simulink model "ModeAdjust"  (R2018b)
settings: Solver=FixedStepDiscrete  StartTime=0.0  StopTime=inf  FixedStep=0.01  RelTol=1e-3
undefined symbols (not defined in the file or in its folder): IfKeSMSbSeatMovBkRclnEnable_Val, IfKeSMSbSeatMovFrwdBkwdEnable_Val, IfKeSMSbSeatMovFtrstEnable_Val, IfKeSMSbSeatMovHdrstFrwdBkwdEnable_Val, IfKeSMSbSeatMovHdUpwdDnwdEnable_Val, IfKeSMSbSeatMovLgrstEnable_Val, IfKeSMSbSeatMovLtwdRtwdEnable_Val, IfVeSMSeStNumConfig, KeSMSbArmscreenMovEnable_Val, KeSMSbSeatMovLgrstExpdEnable_Val, KeSMSuFirstRwStBackPosDelta_Val, KeSMSuFirstRwStBackPosTolr_Val, KeSMSuFirstRwStCushFrntPosDelta_Val, KeSMSuFirstRwStCushFrntPosTolr_Val, KeSMSuFirstRwStCushRePosDelta_Val, KeSMSuFirstRwStCushRePosTolr_Val, KeSMSuFirstRwStFootrestPosDelta_Val, KeSMSuFirstRwStFootrestPosTolr_Val, KeSMSuFirstRwStFwdBkwdPosDelta_Val, KeSMSuFirstRwStFwdBkwdPosTolr_Val, KeSMSuMdMotFinshdTm_Val, KeSMSuMdRetryTm1_Val, KeSMSuModeReqDurgTm_Val, KeSMSuSecRwStArmTochPosDelta_Val, KeSMSuSecRwStArmTochPosTolr_Val, KeSMSuSecRwStBackPosDelta_Val, KeSMSuSecRwStBackPosTolr_Val, KeSMSuSecRwStFtrstUpwdDnwdPosDelta_Val, KeSMSuSecRwStFtrstUpwdDnwdPosTolr_Val, KeSMSuSecRwStFwdBkwdPosDelta_Val, KeSMSuSecRwStFwdBkwdPosTolr_Val, KeSMSuSecRwStHeadrestFwdBkwdPosDelta_Val, KeSMSuSecRwStHeadrestFwdBkwdPosTolr_Val, KeSMSuSecRwStHeadrestUpwdDwnwdPosDelta_Val, KeSMSuSecRwStHeadrestUpwdDwnwdPosTolr_Val, KeSMSuSecRwStLegrestInOutPosDelta_Val, KeSMSuSecRwStLegrestInOutPosTolr_Val, KeSMSuSecRwStLegrestUpwdDwnwdPosDelta_Val, KeSMSuSecRwStLegrestUpwdDwnwdPosTolr_Val, KeSMSuSecRwStLwdRwdPosDelta_Val, KeSMSuSecRwStLwdRwdPosTolr_Val, KeSMSuSecRwStVIPFtrstRefAngle_Val, KeSMSuThirdRwStFwdBkwdPosDelta_Val, KeSMSuThirdRwStFwdBkwdPosTolr_Val, KeSMSuThrdRwCushFoldPosDelta_Val, KeSMSuThrdRwCushFoldPosTolr_Val, KeSMSuThrdRwStBackPosDelta_Val, KeSMSuThrdRwStBackPosTolr_Val, KeSMSw4SLegrstCloseMdSecRwLtStFtrstUpwdDnwdPos_Val, KeSMSw4SLegrstCloseMdSecRwLtStFtrstUpwdDnwdPosMax_Val, KeSMSw4SLegrstCloseMdSecRwLtStFtrstUpwdDnwdPosMin_Val, KeSMSw4SLegrstCloseMdSecRwLtStLgrstOtwdInwdPos_Val, KeSMSw4SLegrstCloseMdSecRwLtStLgrstOtwdInwdPosMax_Val, KeSMSw4SLegrstCloseMdSecRwLtStLgrstOtwdInwdPosMin_Val, KeSMSw4SLegrstCloseMdSecRwLtStLgrstUpwdDnwdPos_Val, KeSMSw4SLegrstCloseMdSecRwLtStLgrstUpwdDnwdPosMax_Val, KeSMSw4SLegrstCloseMdSecRwLtStLgrstUpwdDnwdPosMin_Val, KeSMSw4SLegrstCloseMdSecRwRtStFtrstUpwdDnwdPos_Val, KeSMSw4SLegrstCloseMdSecRwRtStFtrstUpwdDnwdPosMax_Val, KeSMSw4SLegrstCloseMdSecRwRtStFtrstUpwdDnwdPosMin_Val ... (+1138)
libraries: Lib x401
(part 14 of 35)

== system ModeAdjust/ModeAdjustRunnable_sys/ModeAdjust/ArrivedAtTargetPosChk/INTMR ==
  SecRwLtStsPoss : Inport
  SecRwRtStPoss : Inport  Port=2
  ModeStCalib : Inport  Port=3
  StConfig : Inport  Port=4
  SecRwLtStsPossV : Inport  Port=5
  SecRwRtStPossV : Inport  Port=6
  PosDeltaCalib : Inport  Port=7
  Bus Selector : BusSelector  OutputSignals=Calib_Drv,Calib_Pass,Calib_2L,Calib_2R,Calib_3L,Calib_3R
  Bus Selector1 : BusSelector  OutputSignals=DrvStConfig,PassStConfig,SecRwLtStConfig,SecRwRtStConfig,ThdRwLtStConfig,ThdRwRtStConfig
  Logical Operator : Logic  AllPortsSameDT=off  OutDataTypeStr=boolean
  R2Lt : Subsystem
  R2Rt : Subsystem
  isINTMArrivedAtTargetPos : Outport
  wires:
  SecRwRtStPossV/1 -> R2Rt/4(SecRwRtStPossV)
  SecRwLtStsPossV/1 -> R2Lt/4(SecRwLtStPossV)
  [R2RtST_ArrivedTarPos] -> Logical Operator/2
  [R2LtST_ArrivedTarPos] -> Logical Operator/1
  Logical Operator/1 -> isINTMArrivedAtTargetPos/1
  R2Lt/1(R2Lt_ArrivedTarPos) -> [R2LtST_ArrivedTarPos]
  R2Rt/1(R2Rt_ArrivedTarPos) -> [R2RtST_ArrivedTarPos]
  SecRwLtStsPoss/1 -> R2Rt/5(SecRwLtStsPoss), R2Lt/1(SecRwLtStsPoss)
  SecRwRtStPoss/1 -> R2Rt/1(SecRwRtStPoss)
  Bus Selector/6 -> [ModeStCalib_3R]  "<Calib_3R>"
  Bus Selector/4 -> [ModeStCalib_2R]  "<Calib_2R>"
  Bus Selector/1 -> [ModeStCalib_Drv]  "<Calib_Drv>"
  Bus Selector/3 -> [ModeStCalib_2L]  "<Calib_2L>"
  Bus Selector/5 -> [ModeStCalib_3L]  "<Calib_3L>"
  Bus Selector/2 -> [ModeStCalib_Pass]  "<Calib_Pass>"
  ModeStCalib/1 -> Bus Selector/1
  [ModeStCalib_2R] -> R2Rt/2(ModeStCalib_2R)
  [ModeStCalib_2L] -> R2Lt/2(ModeStCalib_2L)
  Bus Selector1/6 -> [ThdRwRtStConfig]  "<ThdRwRtStConfig>"
  Bus Selector1/1 -> [DrvStConfig]  "<DrvStConfig>"
  Bus Selector1/3 -> [SecRwLtStConfig]  "<SecRwLtStConfig>"
  Bus Selector1/4 -> [SecRwRtStConfig]  "<SecRwRtStConfig>"
  StConfig/1 -> Bus Selector1/1
  Bus Selector1/2 -> [PassStConfig]  "<PassStConfig>"
  Bus Selector1/5 -> [ThdRwLtStConfig]  "<ThdRwLtStConfig>"
  [SecRwLtStConfig] -> R2Lt/3(StConfig)
  [SecRwRtStConfig] -> R2Rt/3(StConfig)
  PosDeltaCalib/1 -> [PosDeltaCalib]
  [PosDeltaCalib] -> R2Lt/5(PosDeltaCalib)
  [PosDeltaCalib] -> R2Rt/6(PosDeltaCalib)

== system ModeAdjust/ModeAdjustRunnable_sys/ModeAdjust/ArrivedAtTargetPosChk/LgrstClose ==
  SecRwLtStsPoss : Inport
  SecRwRtStPoss : Inport  Port=2
  ModeStCalib : Inport  Port=3
  StConfig : Inport  Port=4
  SecRwLtStsPoss4s : Inport  Port=5
  SecRwRtStsPoss4s : Inport  Port=6
  StConfig4s : Inport  Port=7
  SecRwLtStsPossV : Inport  Port=8
  SecRwRtStPossV : Inport  Port=9
  SecRwLtStsPoss4sV : Inport  Port=10
  SecRwRtStsPoss4sV : Inport  Port=11
  PosDeltaCalib : Inport  Port=12
  Bus Selector : BusSelector  OutputSignals=Calib_Drv,Calib_Pass,Calib_2L,Calib_2R,Calib_3L,Calib_3R,Calib_2L4s,Calib_2R4s
  Bus Selector1 : BusSelector  OutputSignals=DrvStConfig,PassStConfig,SecRwLtStConfig,SecRwRtStConfig,ThdRwLtStConfig,ThdRwRtStConfig
  Bus Selector5 : BusSelector  OutputSignals=SecRwLtStConfig,SecRwRtStConfig
  R2Lt : Subsystem
  R2Rt : Subsystem
  isLfRecoveryArrivedAtTargetPos : Outport
  isRtRecoveryArrivedAtTargetPos : Outport  Port=2
  wires:
  SecRwLtStsPoss4sV/1 -> R2Lt/7(SecRwLtStPossV4s)
  SecRwRtStsPoss4sV/1 -> R2Rt/7(PosV4s)
  SecRwRtStPossV/1 -> R2Rt/6(SecRwRtStPossV)
  SecRwLtStsPossV/1 -> R2Lt/6(SecRwLtStPossV)
  [R2LtST_ArrivedTarPos] -> isLfRecoveryArrivedAtTargetPos/1
  R2Lt/1(R2Lt_ArrivedTarPos) -> [R2LtST_ArrivedTarPos]
  R2Rt/1(R2Lt_ArrivedTarPos) -> [R2RtST_ArrivedTarPos]
  SecRwLtStsPoss/1 -> R2Lt/1(SecRwLtStsPoss)
  SecRwRtStPoss/1 -> R2Rt/1(SecRwLtStsPoss)
  [R2RtST_ArrivedTarPos] -> isRtRecoveryArrivedAtTargetPos/1
  Bus Selector/6 -> [ModeStCalib_3R]  "<Calib_3R>"
  Bus Selector/4 -> [ModeStCalib_2R]  "<Calib_2R>"
  Bus Selector/1 -> [ModeStCalib_Drv]  "<Calib_Drv>"
  Bus Selector/3 -> [ModeStCalib_2L]  "<Calib_2L>"
  Bus Selector/5 -> [ModeStCalib_3L]  "<Calib_3L>"
  Bus Selector/2 -> [ModeStCalib_Pass]  "<Calib_Pass>"
  ModeStCalib/1 -> Bus Selector/1
  [Calib_2R4s] -> R2Rt/2(ModeStCalib_2L)
  [Calib_2L4s] -> R2Lt/2(ModeStCalib_2L)
  Bus Selector1/6 -> [ThdRwRtStConfig]  "<ThdRwRtStConfig>"
  Bus Selector1/1 -> [DrvStConfig]  "<DrvStConfig>"
  Bus Selector1/3 -> [SecRwLtStConfig]  "<SecRwLtStConfig>"
  Bus Selector1/4 -> [SecRwRtStConfig]  "<SecRwRtStConfig>"
  StConfig/1 -> Bus Selector1/1
  Bus Selector1/2 -> [PassStConfig]  "<PassStConfig>"
  Bus Selector1/5 -> [ThdRwLtStConfig]  "<ThdRwLtStConfig>"
  [SecRwLtStConfig] -> R2Lt/3(StConfig)
  [SecRwRtStConfig] -> R2Rt/3(StConfig)
  Bus Selector/8 -> [Calib_2R4s]  "<Calib_2R4s>"
  Bus Selector/7 -> [Calib_2L4s]  "<Calib_2L4s>"
  SecRwLtStsPoss4s/1 -> R2Lt/4(SecRwLtStsPoss4s)
  SecRwRtStsPoss4s/1 -> R2Rt/4(SecRwLtStsPoss4s)
  StConfig4s/1 -> Bus Selector5/1
  Bus Selector5/1 -> [SecRwLtStConfig4s]  "<SecRwLtStConfig>"
  Bus Selector5/2 -> [SecRwRtStConfig4s]  "<SecRwRtStConfig>"
  [SecRwLtStConfig4s] -> R2Lt/5(StConfig4s)
  [SecRwRtStConfig4s] -> R2Rt/5(StConfig4s)
  PosDeltaCalib/1 -> [PosDeltaCalib]
  [PosDeltaCalib] -> R2Lt/8(PosDeltaCalib)
  [PosDeltaCalib] -> R2Rt/8(PosDeltaCalib)

== system ModeAdjust/ModeAdjustRunnable_sys/ModeAdjust/ArrivedAtTargetPosChk/LgrstOpen ==
  SecRwLtStsPoss : Inport
  SecRwRtStPoss : Inport  Port=2
  ModeStCalib : Inport  Port=3
  StConfig : Inport  Port=4
  SecRwLtStsPoss4s : Inport  Port=5
  SecRwRtStsPoss4s : Inport  Port=6
  StConfig4s : Inport  Port=7
  SecRwLtStsPossV : Inport  Port=8
  SecRwRtStPossV : Inport  Port=9
  SecRwLtStsPoss4sV : Inport  Port=10
  SecRwRtStsPoss4sV : Inport  Port=11
  PosDeltaCalib : Inport  Port=12
  Bus Selector : BusSelector  OutputSignals=Calib_Drv,Calib_Pass,Calib_2L,Calib_2R,Calib_3L,Calib_3R,Calib_2L4s,Calib_2R4s
  Bus Selector1 : BusSelector  OutputSignals=DrvStConfig,PassStConfig,SecRwLtStConfig,SecRwRtStConfig,ThdRwLtStConfig,ThdRwRtStConfig
  Bus Selector5 : BusSelector  OutputSignals=SecRwLtStConfig,SecRwRtStConfig
  R2Lt : Subsystem
  R2Rt : Subsystem
  isLfRecoveryArrivedAtTargetPos : Outport
  isRtRecoveryArrivedAtTargetPos : Outport  Port=2
  wires:
  [SecRwRtStConfig4s] -> R2Rt/5(StConfig4s)
  [SecRwLtStConfig4s] -> R2Lt/5(StConfig4s)
  Bus Selector5/2 -> [SecRwRtStConfig4s]  "<SecRwRtStConfig>"
  Bus Selector5/1 -> [SecRwLtStConfig4s]  "<SecRwLtStConfig>"
  StConfig4s/1 -> Bus Selector5/1
  SecRwRtStsPoss4s/1 -> R2Rt/4(SecRwLtStsPoss4s)
  SecRwLtStsPoss4s/1 -> R2Lt/4(SecRwLtStsPoss4s)
  Bus Selector/7 -> [Calib_2L4s]  "<Calib_2L4s>"
  Bus Selector/8 -> [Calib_2R4s]  "<Calib_2R4s>"
  [SecRwRtStConfig] -> R2Rt/3(StConfig)
  [SecRwLtStConfig] -> R2Lt/3(StConfig)
  Bus Selector1/5 -> [ThdRwLtStConfig]  "<ThdRwLtStConfig>"
  Bus Selector1/2 -> [PassStConfig]  "<PassStConfig>"
  StConfig/1 -> Bus Selector1/1
  Bus Selector1/4 -> [SecRwRtStConfig]  "<SecRwRtStConfig>"
  Bus Selector1/3 -> [SecRwLtStConfig]  "<SecRwLtStConfig>"
  Bus Selector1/1 -> [DrvStConfig]  "<DrvStConfig>"
  Bus Selector1/6 -> [ThdRwRtStConfig]  "<ThdRwRtStConfig>"
  [Calib_2L4s] -> R2Lt/2(ModeStCalib_2L)
  [Calib_2R4s] -> R2Rt/2(ModeStCalib_2L)
  ModeStCalib/1 -> Bus Selector/1
  Bus Selector/2 -> [ModeStCalib_Pass]  "<Calib_Pass>"
  Bus Selector/5 -> [ModeStCalib_3L]  "<Calib_3L>"
  Bus Selector/3 -> [ModeStCalib_2L]  "<Calib_2L>"
  Bus Selector/1 -> [ModeStCalib_Drv]  "<Calib_Drv>"
  Bus Selector/4 -> [ModeStCalib_2R]  "<Calib_2R>"
  Bus Selector/6 -> [ModeStCalib_3R]  "<Calib_3R>"
  [R2RtST_ArrivedTarPos] -> isRtRecoveryArrivedAtTargetPos/1
  SecRwRtStPoss/1 -> R2Rt/1(SecRwLtStsPoss)
  SecRwLtStsPoss/1 -> R2Lt/1(SecRwLtStsPoss)
  R2Rt/1(R2Lt_ArrivedTarPos) -> [R2RtST_ArrivedTarPos]
  R2Lt/1(R2Lt_ArrivedTarPos) -> [R2LtST_ArrivedTarPos]
  [R2LtST_ArrivedTarPos] -> isLfRecoveryArrivedAtTargetPos/1
  SecRwLtStsPossV/1 -> R2Lt/6(SecRwLtStPossV)
  SecRwLtStsPoss4sV/1 -> R2Lt/7(SecRwLtStPossV4s)
  SecRwRtStPossV/1 -> R2Rt/6(SecRwRtStPossV)
  SecRwRtStsPoss4sV/1 -> R2Rt/7(PosV4s)
  PosDeltaCalib/1 -> [PosDeltaCalib]
  [PosDeltaCalib] -> R2Lt/8(PosDeltaCalib)
  [PosDeltaCalib] -> R2Rt/8(PosDeltaCalib)

== system ModeAdjust/ModeAdjustRunnable_sys/ModeAdjust/ArrivedAtTargetPosChk/Lug ==
  ThdRwLtStPoss : Inport
  ThdRwRtStPoss : Inport  Port=2
  ModeStCalib : Inport  Port=3
  is6s : Inport  Port=4
  StConfig : Inport  Port=5
  IfVeSMSbThdRwLtStFrwdCmdSrv_Val_read : Inport  Port=6
  IfVeSMSbThdRwRtStFrwdCmdSrv_Val_read : Inport  Port=7
  ThdRwLtStPossV : Inport  Port=8
  ThdRwRtStPossV : Inport  Port=9
  PosDeltaCalib : Inport  Port=10
  Bus Selector : BusSelector  OutputSignals=Calib_Drv,Calib_Pass,Calib_2L,Calib_2R,Calib_3L,Calib_3R
  Bus Selector1 : BusSelector  OutputSignals=DrvStConfig,PassStConfig,SecRwLtStConfig,SecRwRtStConfig,ThdRwLtStConfig,ThdRwRtStConfig
  R3Lt : Subsystem
  R3Rt : Subsystem
  Subsystem1 : Subsystem
  isLfLugArrivedAtTargetPos : Outport
  isRtLugArrivedAtTargetPos : Outport  Port=2
  wires:
  ThdRwRtStPoss/1 -> R3Rt/1(ThdRwRtStPoss)
  ThdRwLtStPoss/1 -> R3Lt/1(ThdRwLtStPoss)
  R3Rt/1(R3Rt_ArrivedTarPos) -> [R3RtST_ArrivedTarPos]
  R3Lt/1(R3Lt_ArrivedTarPos) -> [R3LtST_ArrivedTarPos]
  Subsystem1/1(Md_L_MvDoneOK) -> isLfLugArrivedAtTargetPos/1
  [R3LtST_ArrivedTarPos] -> Subsystem1/1(Left_inport)
  [R3RtST_ArrivedTarPos] -> Subsystem1/2(Right_inport)
  Subsystem1/2(Md_R_MvDoneOK) -> isRtLugArrivedAtTargetPos/1
  Bus Selector/6 -> [ModeStCalib_3R]  "<Calib_3R>"
  Bus Selector/4 -> [ModeStCalib_2R]  "<Calib_2R>"
  Bus Selector/1 -> [ModeStCalib_Drv]  "<Calib_Drv>"
  Bus Selector/3 -> [ModeStCalib_2L]  "<Calib_2L>"
  Bus Selector/5 -> [ModeStCalib_3L]  "<Calib_3L>"
  Bus Selector/2 -> [ModeStCalib_Pass]  "<Calib_Pass>"
  ModeStCalib/1 -> Bus Selector/1
  [ModeStCalib_3L] -> R3Lt/2(ModeStCalib_3L)
  [ModeStCalib_3R] -> R3Rt/2(ModeStCalib_3R)
  is6s/1 -> [is6s]
  [is6s] -> R3Lt/3(is6s)
  [is6s] -> R3Rt/3(is6s)
  Bus Selector1/6 -> [ThdRwRtStConfig]  "<ThdRwRtStConfig>"
  Bus Selector1/1 -> [DrvStConfig]  "<DrvStConfig>"
  Bus Selector1/3 -> [SecRwLtStConfig]  "<SecRwLtStConfig>"
  Bus Selector1/4 -> [SecRwRtStConfig]  "<SecRwRtStConfig>"
  StConfig/1 -> Bus Selector1/1
  Bus Selector1/2 -> [PassStConfig]  "<PassStConfig>"
  Bus Selector1/5 -> [ThdRwLtStConfig]  "<ThdRwLtStConfig>"
  [ThdRwLtStConfig] -> R3Lt/4(StConfig)
  [ThdRwRtStConfig] -> R3Rt/4(StConfig)
  IfVeSMSbThdRwLtStFrwdCmdSrv_Val_read/1 -> R3Lt/5(IfVeSMSbThdRwLtStFrwdCmdSrv_Val_read)
  IfVeSMSbThdRwRtStFrwdCmdSrv_Val_read/1 -> R3Rt/5(IfVeSMSbThdRwRtStFrwdCmdSrv_Val_read)
  ThdRwLtStPossV/1 -> R3Lt/6(ThdRwLtStPossV)
  ThdRwRtStPossV/1 -> R3Rt/6(ThdRwRtStPossV)
  PosDeltaCalib/1 -> [PosDeltaCalib]
  [PosDeltaCalib] -> R3Lt/7(PosDeltaCalib)
  [PosDeltaCalib] -> R3Rt/7(PosDeltaCalib)

== system ModeAdjust/ModeAdjustRunnable_sys/ModeAdjust/ArrivedAtTargetPosChk/Ly ==
  SecRwLtStsPoss : Inport
  SecRwRtStPoss : Inport  Port=2
  ModeStCalib : Inport  Port=3
  StConfig : Inport  Port=4
  SecRwLtStsPoss4s : Inport  Port=5
  SecRwRtStsPoss4s : Inport  Port=6
  StConfig4s : Inport  Port=7
  SecRwLtStsPossV : Inport  Port=8
  SecRwRtStPossV : Inport  Port=9
  SecRwLtStsPoss4sV : Inport  Port=10
  SecRwRtStsPoss4sV : Inport  Port=11
  Lt4sHightIndex : Inport  Port=12
  Rt4sHightIndex : Inport  Port=13
  PosDeltaCalib : Inport  Port=14
  Bus Selector : BusSelector  OutputSignals=Calib_Drv,Calib_Pass,Calib_2L,Calib_2R,Calib_3L,Calib_3R,Calib_2L4s,Calib_2R4s
  Bus Selector1 : BusSelector  OutputSignals=DrvStConfig,PassStConfig,SecRwLtStConfig,SecRwRtStConfig,ThdRwLtStConfig,ThdRwRtStConfig
  Bus Selector5 : BusSelector  OutputSignals=SecRwLtStConfig,SecRwRtStConfig
  R2Lt : Subsystem
  R2Rt : Subsystem
  isLfRecoveryArrivedAtTargetPos : Outport
  isRtRecoveryArrivedAtTargetPos : Outport  Port=2
  Calib_Ly4sLAdpt : Outport  Port=3
  Calib_Ly4sRAdpt : Outport  Port=4
  wires:
  [R2LtST_ArrivedTarPos] -> isLfRecoveryArrivedAtTargetPos/1
  R2Lt/1(R2Lt_ArrivedTarPos) -> [R2LtST_ArrivedTarPos]
  R2Rt/1(R2Lt_ArrivedTarPos) -> [R2RtST_ArrivedTarPos]
  SecRwLtStsPoss/1 -> R2Lt/1(SecRwLtStsPoss)
  SecRwRtStPoss/1 -> R2Rt/1(SecRwLtStsPoss)
  [R2RtST_ArrivedTarPos] -> isRtRecoveryArrivedAtTargetPos/1
  Bus Selector/6 -> [ModeStCalib_3R]  "<Calib_3R>"
  Bus Selector/4 -> [ModeStCalib_2R]  "<Calib_2R>"
  Bus Selector/1 -> [ModeStCalib_Drv]  "<Calib_Drv>"
  Bus Selector/3 -> [ModeStCalib_2L]  "<Calib_2L>"
  Bus Selector/5 -> [ModeStCalib_3L]  "<Calib_3L>"
  Bus Selector/2 -> [ModeStCalib_Pass]  "<Calib_Pass>"
  ModeStCalib/1 -> Bus Selector/1
  [Calib_2R4s] -> R2Rt/2(ModeStCalib_2L)
  [Calib_2L4s] -> R2Lt/2(ModeStCalib_2L)
  Bus Selector1/6 -> [ThdRwRtStConfig]  "<ThdRwRtStConfig>"
  Bus Selector1/1 -> [DrvStConfig]  "<DrvStConfig>"
  Bus Selector1/3 -> [SecRwLtStConfig]  "<SecRwLtStConfig>"
  Bus Selector1/4 -> [SecRwRtStConfig]  "<SecRwRtStConfig>"
  StConfig/1 -> Bus Selector1/1
  Bus Selector1/2 -> [PassStConfig]  "<PassStConfig>"
  Bus Selector1/5 -> [ThdRwLtStConfig]  "<ThdRwLtStConfig>"
  [SecRwLtStConfig] -> R2Lt/3(StConfig)
  [SecRwRtStConfig] -> R2Rt/3(StConfig)
  Bus Selector/8 -> [Calib_2R4s]  "<Calib_2R4s>"
  Bus Selector/7 -> [Calib_2L4s]  "<Calib_2L4s>"
  SecRwLtStsPoss4s/1 -> R2Lt/4(SecRwLtStsPoss4s)
  SecRwRtStsPoss4s/1 -> R2Rt/4(SecRwLtStsPoss4s)
  StConfig4s/1 -> Bus Selector5/1
  Bus Selector5/1 -> [SecRwLtStConfig4s]  "<SecRwLtStConfig>"
  Bus Selector5/2 -> [SecRwRtStConfig4s]  "<SecRwRtStConfig>"
  [SecRwLtStConfig4s] -> R2Lt/5(StConfig4s)
  [SecRwRtStConfig4s] -> R2Rt/5(StConfig4s)
  SecRwLtStsPoss4sV/1 -> R2Lt/7(SecRwLtStPossV4s)
  SecRwRtStsPoss4sV/1 -> R2Rt/7(PosV4s)
  SecRwLtStsPossV/1 -> R2Lt/6(SecRwLtStPossV)
  SecRwRtStPossV/1 -> R2Rt/6(SecRwRtStPossV)
  Lt4sHightIndex/1 -> R2Lt/8(Lt4sHightIndex)
  Rt4sHightIndex/1 -> R2Rt/8(Rt4sHightIndex)
  R2Lt/2(Calib_Ly4sLAdpt) -> Calib_Ly4sLAdpt/1
  R2Rt/2(Calib_Ly4sRAdpt) -> Calib_Ly4sRAdpt/1
  PosDeltaCalib/1 -> [PosDeltaCalib]
  [PosDeltaCalib] -> R2Lt/9(PosDeltaCalib)
  [PosDeltaCalib] -> R2Rt/9(PosDeltaCalib)

== system ModeAdjust/ModeAdjustRunnable_sys/ModeAdjust/ArrivedAtTargetPosChk/Recovery ==
  SecRwLtStsPoss : Inport
  SecRwRtStPoss : Inport  Port=2
  ModeStCalib : Inport  Port=3
  StConfig : Inport  Port=4
  DrvCurPos : Inport  Port=5
  PassStPoss : Inport  Port=6
  DrvCurPosV : Inport  Port=7
  PassStPossV : Inport  Port=8
  SecRwLtStsPossV : Inport  Port=9
  SecRwRtStPossV : Inport  Port=10
  PosDeltaCalib : Inport  Port=11
  Bus Selector : BusSelector  OutputSignals=Calib_Drv,Calib_Pass,Calib_2L,Calib_2R,Calib_3L,Calib_3R
  Bus Selector1 : BusSelector  OutputSignals=DrvStConfig,PassStConfig,SecRwLtStConfig,SecRwRtStConfig,ThdRwLtStConfig,ThdRwRtStConfig
  Drv : Subsystem
  Logical Operator : Logic  AllPortsSameDT=off  OutDataTypeStr=boolean
  Logical Operator1 : Logic  AllPortsSameDT=off  OutDataTypeStr=boolean
  Pass : Subsystem
  R2Lt : Subsystem
  R2Rt : Subsystem
  isLfRecoveryArrivedAtTargetPos : Outport
  isRtRecoveryArrivedAtTargetPos : Outport  Port=2
  wires:
  Logical Operator/1 -> isLfRecoveryArrivedAtTargetPos/1
  R2Lt/1(R2Lt_ArrivedTarPos) -> [R2LtST_ArrivedTarPos]
  R2Rt/1(R2Rt_ArrivedTarPos) -> [R2RtST_ArrivedTarPos]
  SecRwLtStsPoss/1 -> R2Lt/1(SecRwLtStsPoss)
  SecRwRtStPoss/1 -> R2Rt/1(SecRwRtStPoss)
  Logical Operator1/1 -> isRtRecoveryArrivedAtTargetPos/1
  Bus Selector/6 -> [ModeStCalib_3R]  "<Calib_3R>"
  Bus Selector/4 -> [ModeStCalib_2R]  "<Calib_2R>"
  Bus Selector/1 -> [ModeStCalib_Drv]  "<Calib_Drv>"
  Bus Selector/3 -> [ModeStCalib_2L]  "<Calib_2L>"
  Bus Selector/5 -> [ModeStCalib_3L]  "<Calib_3L>"
  Bus Selector/2 -> [ModeStCalib_Pass]  "<Calib_Pass>"
  ModeStCalib/1 -> Bus Selector/1
  [ModeStCalib_2R] -> R2Rt/2(ModeStCalib_2R)
  [ModeStCalib_2L] -> R2Lt/2(ModeStCalib_2L)
  Bus Selector1/6 -> [ThdRwRtStConfig]  "<ThdRwRtStConfig>"
  Bus Selector1/1 -> [DrvStConfig]  "<DrvStConfig>"
  Bus Selector1/3 -> [SecRwLtStConfig]  "<SecRwLtStConfig>"
  Bus Selector1/4 -> [SecRwRtStConfig]  "<SecRwRtStConfig>"
  StConfig/1 -> Bus Selector1/1
  Bus Selector1/2 -> [PassStConfig]  "<PassStConfig>"
  Bus Selector1/5 -> [ThdRwLtStConfig]  "<ThdRwLtStConfig>"
  [SecRwLtStConfig] -> R2Lt/3(StConfig)
  [SecRwRtStConfig] -> R2Rt/3(StConfig)
  Drv/1(Drv_ArrivedTarPos) -> [DrvST_ArrivedTarPos]
  [DrvStConfig] -> Drv/3(StConfig)
  DrvCurPos/1 -> Drv/1(DrvCurPos)
  [ModeStCalib_Drv] -> Drv/2(ModeStCalib_Drv)
  Pass/1(Pass_ArrivedTarPos) -> [Pass_ArrivedTarPos]
  [ModeStCalib_Pass] -> Pass/2(ModeStCalib_Pass)
  PassStPoss/1 -> Pass/1(PassStPoss)
  [PassStConfig] -> Pass/3(StConfig)
  [R2LtST_ArrivedTarPos] -> Logical Operator/1
  [DrvST_ArrivedTarPos] -> Logical Operator/2
  [R2RtST_ArrivedTarPos] -> Logical Operator1/1
  [Pass_ArrivedTarPos] -> Logical Operator1/2
  DrvCurPosV/1 -> Drv/4(DrvCurPosV)
  PassStPossV/1 -> Pass/4(PassStPossV)
  SecRwLtStsPossV/1 -> R2Lt/4(SecRwLtStPossV)
  SecRwRtStPossV/1 -> R2Rt/4(SecRwRtStPossV)
  PosDeltaCalib/1 -> [PosDeltaCalib]
  [PosDeltaCalib] -> Drv/5(PosDeltaCalib)
  [PosDeltaCalib] -> Pass/5(PosDeltaCalib)
  [PosDeltaCalib] -> R2Lt/5(PosDeltaCalib)
  [PosDeltaCalib] -> R2Rt/5(PosDeltaCalib)

== system ModeAdjust/ModeAdjustRunnable_sys/ModeAdjust/ArrivedAtTargetPosChk/Recovery4s ==
  SecRwLtStsPoss : Inport
  SecRwRtStPoss : Inport  Port=2
  ModeStCalib : Inport  Port=3
  StConfig : Inport  Port=4
  SecRwLtStsPoss4s : Inport  Port=5
  SecRwRtStsPoss4s : Inport  Port=6
  StConfig4s : Inport  Port=7
  SecRwLtStsPossV : Inport  Port=8
  SecRwRtStPossV : Inport  Port=9
  SecRwLtStsPoss4sV : Inport  Port=10
  SecRwRtStsPoss4sV : Inport  Port=11
  Lt4sHightIndex : Inport  Port=12
  Rt4sHightIndex : Inport  Port=13
  PosDeltaCalib : Inport  Port=14
  Bus Selector : BusSelector  OutputSignals=Calib_Drv,Calib_Pass,Calib_2L,Calib_2R,Calib_3L,Calib_3R,Calib_2L4s,Calib_2R4s
  Bus Selector1 : BusSelector  OutputSignals=DrvStConfig,PassStConfig,SecRwLtStConfig,SecRwRtStConfig,ThdRwLtStConfig,ThdRwRtStConfig
  Bus Selector5 : BusSelector  OutputSignals=SecRwLtStConfig,SecRwRtStConfig
  R2Lt : Subsystem
  R2Rt : Subsystem
  isLfRecoveryArrivedAtTargetPos : Outport
  isRtRecoveryArrivedAtTargetPos : Outport  Port=2
  Calib_Recoery4sLAdpt : Outport  Port=3
  Calib_Recoery4sRAdpt : Outport  Port=4
  wires:
  [SecRwRtStConfig4s] -> R2Rt/5(StConfig4s)
  [SecRwLtStConfig4s] -> R2Lt/5(StConfig4s)
  Bus Selector5/2 -> [SecRwRtStConfig4s]  "<SecRwRtStConfig>"
  Bus Selector5/1 -> [SecRwLtStConfig4s]  "<SecRwLtStConfig>"
  StConfig4s/1 -> Bus Selector5/1
  SecRwRtStsPoss4s/1 -> R2Rt/4(SecRwLtStsPoss4s)
  SecRwLtStsPoss4s/1 -> R2Lt/4(SecRwLtStsPoss4s)
  Bus Selector/7 -> [Calib_2L4s]  "<Calib_2L4s>"
  Bus Selector/8 -> [Calib_2R4s]  "<Calib_2R4s>"
  [SecRwRtStConfig] -> R2Rt/3(StConfig)
  [SecRwLtStConfig] -> R2Lt/3(StConfig)
  Bus Selector1/5 -> [ThdRwLtStConfig]  "<ThdRwLtStConfig>"
  Bus Selector1/2 -> [PassStConfig]  "<PassStConfig>"
  StConfig/1 -> Bus Selector1/1
  Bus Selector1/4 -> [SecRwRtStConfig]  "<SecRwRtStConfig>"
  Bus Selector1/3 -> [SecRwLtStConfig]  "<SecRwLtStConfig>"
  Bus Selector1/1 -> [DrvStConfig]  "<DrvStConfig>"
  Bus Selector1/6 -> [ThdRwRtStConfig]  "<ThdRwRtStConfig>"
  [Calib_2L4s] -> R2Lt/2(ModeStCalib_2L)
  [Calib_2R4s] -> R2Rt/2(ModeStCalib_2L)
  ModeStCalib/1 -> Bus Selector/1
  Bus Selector/2 -> [ModeStCalib_Pass]  "<Calib_Pass>"
  Bus Selector/5 -> [ModeStCalib_3L]  "<Calib_3L>"
  Bus Selector/3 -> [ModeStCalib_2L]  "<Calib_2L>"
  Bus Selector/1 -> [ModeStCalib_Drv]  "<Calib_Drv>"
  Bus Selector/4 -> [ModeStCalib_2R]  "<Calib_2R>"
  Bus Selector/6 -> [ModeStCalib_3R]  "<Calib_3R>"
  [R2RtST_ArrivedTarPos] -> isRtRecoveryArrivedAtTargetPos/1
  SecRwRtStPoss/1 -> R2Rt/1(SecRwLtStsPoss)
  SecRwLtStsPoss/1 -> R2Lt/1(SecRwLtStsPoss)
  R2Rt/1(R2Lt_ArrivedTarPos) -> [R2RtST_ArrivedTarPos]
  R2Lt/1(R2Lt_ArrivedTarPos) -> [R2LtST_ArrivedTarPos]
  [R2LtST_ArrivedTarPos] -> isLfRecoveryArrivedAtTargetPos/1
  SecRwLtStsPossV/1 -> R2Lt/6(SecRwLtStPossV)
  SecRwRtStPossV/1 -> R2Rt/6(SecRwRtStPossV)
  SecRwRtStsPoss4sV/1 -> R2Rt/7(PosV4s)
  SecRwLtStsPoss4sV/1 -> R2Lt/7(SecRwLtStPossV4s)
  Lt4sHightIndex/1 -> R2Lt/8(Lt4sHightIndex)
  Rt4sHightIndex/1 -> R2Rt/8(Rt4sHightIndex)
  R2Lt/2(Calib_Recoery4sLAdpt) -> Calib_Recoery4sLAdpt/1
  R2Rt/2(Calib_Recoery4sRAdpt) -> Calib_Recoery4sRAdpt/1
  PosDeltaCalib/1 -> [PosDeltaCalib]
  [PosDeltaCalib] -> R2Lt/9(PosDeltaCalib)
  [PosDeltaCalib] -> R2Rt/9(PosDeltaCalib)

== system ModeAdjust/ModeAdjustRunnable_sys/ModeAdjust/ArrivedAtTargetPosChk/VIP ==
  SecRwLtStsPoss : Inport
  SecRwRtStPoss : Inport  Port=2
  ThdRwLtStPoss : Inport  Port=3
  ThdRwRtStPoss : Inport  Port=4
  ModeStCalib : Inport  Port=5
  is6s : Inport  Port=6
  StConfig : Inport  Port=7
  DrvCurPos : Inport  Port=8
  PassStPoss : Inport  Port=9
  DrvCurPosV : Inport  Port=10
  PassStPossV : Inport  Port=11
  SecRwLtStsPossV : Inport  Port=12
  SecRwRtStPossV : Inport  Port=13
  ThdRwLtStPossV : Inport  Port=14
  ThdRwRtStPossV : Inport  Port=15
  PosDeltaCalib : Inport  Port=16
  Bus Selector : BusSelector  OutputSignals=Calib_Drv,Calib_Pass,Calib_2L,Calib_2R,Calib_3L,Calib_3R
  Bus Selector1 : BusSelector  OutputSignals=DrvStConfig,PassStConfig,SecRwLtStConfig,SecRwRtStConfig,ThdRwLtStConfig,ThdRwRtStConfig
  Drv : Subsystem
  Logical Operator1 : Logic  Inputs=3  AllPortsSameDT=off  OutDataTypeStr=boolean
  Logical Operator3 : Logic  Operator=OR  AllPortsSameDT=off  OutDataTypeStr=boolean
  Logical Operator7 : Logic  Inputs=4  AllPortsSameDT=off  OutDataTypeStr=boolean
  Pass : Subsystem
  R2Lt : Subsystem
  R2Rt : Subsystem
  R3Lt : Subsystem
  R3Rt : Subsystem
  isLfVipArrivedAtTargetPos : Outport
  isRtVipArrivedAtTargetPos : Outport  Port=2
  Drv_FtUpwdDnwdPosTrgt : Outport  Port=3
  PassSt_FtUpwdDnwdPosTrgt : Outport  Port=4
  wires:
  SecRwRtStPoss/1 -> R2Rt/1(SecRwRtStPoss)
  ThdRwRtStPoss/1 -> R3Rt/1(ThdRwRtStPoss)
  ThdRwLtStPoss/1 -> R3Lt/1(ThdRwLtStPoss)
  SecRwLtStsPoss/1 -> R2Lt/1(SecRwLtStsPoss)
  R3Rt/1(R3Rt_ArrivedTarPos) -> [R3RtST_ArrivedTarPos]
  R3Lt/1(R3Lt_ArrivedTarPos) -> [R3LtST_ArrivedTarPos]
  R2Rt/1(R2Rt_ArrivedTarPos) -> [R2RtST_ArrivedTarPos]
  R2Lt/1(R2Lt_ArrivedTarPos) -> [R2LtST_ArrivedTarPos]
  [R2LtST_ArrivedTarPos] -> Logical Operator1/1  "LfVip_R2LtST_ArrivedTarPos"
  [R3LtST_ArrivedTarPos] -> Logical Operator1/2  "LfVip_R3LtST_ArrivedTarPos"
  [R3RtST_ArrivedTarPos] -> Logical Operator7/2  "RtVip_R3RtST_ArrivedTarPos"
  [R2RtST_ArrivedTarPos] -> Logical Operator7/1  "RtVip_R2RtST_ArrivedTarPos"
  Logical Operator1/1 -> isLfVipArrivedAtTargetPos/1
  Logical Operator7/1 -> isRtVipArrivedAtTargetPos/1
  Bus Selector/6 -> [ModeStCalib_3R]  "<Calib_3R>"
  Bus Selector/4 -> [ModeStCalib_2R]  "<Calib_2R>"
  Bus Selector/1 -> [ModeStCalib_Drv]  "<Calib_Drv>"
  Bus Selector/3 -> [ModeStCalib_2L]  "<Calib_2L>"
  Bus Selector/5 -> [ModeStCalib_3L]  "<Calib_3L>"
  Bus Selector/2 -> [ModeStCalib_Pass]  "<Calib_Pass>"
  ModeStCalib/1 -> Bus Selector/1
  [ModeStCalib_2L] -> R2Lt/2(ModeStCalib_2L)
  [ModeStCalib_2R] -> R2Rt/2(ModeStCalib_2R)
  [ModeStCalib_3L] -> R3Lt/2(ModeStCalib_3L)
  [ModeStCalib_3R] -> R3Rt/2(ModeStCalib_3R)
  is6s/1 -> [is6s]
  Bus Selector1/6 -> [ThdRwRtStConfig]  "<ThdRwRtStConfig>"
  Bus Selector1/1 -> [DrvStConfig]  "<DrvStConfig>"
  Bus Selector1/3 -> [SecRwLtStConfig]  "<SecRwLtStConfig>"
  Bus Selector1/4 -> [SecRwRtStConfig]  "<SecRwRtStConfig>"
  StConfig/1 -> Bus Selector1/1
  Bus Selector1/2 -> [PassStConfig]  "<PassStConfig>"
  Bus Selector1/5 -> [ThdRwLtStConfig]  "<ThdRwLtStConfig>"
  [SecRwLtStConfig] -> R2Lt/3(StConfig)
  [SecRwRtStConfig] -> R2Rt/3(StConfig)
  [ThdRwLtStConfig] -> R3Lt/3(StConfig)
  [ThdRwRtStConfig] -> R3Rt/3(StConfig)
  [is6s] -> Logical Operator3/2
  Logical Operator3/1 -> Logical Operator7/3  "RtVip_R3LtST_ArrivedTarPos"
  [R3LtST_ArrivedTarPos] -> Logical Operator3/1
  [PassStConfig] -> Pass/3(StConfig)
  PassStPoss/1 -> Pass/1(PassStPoss)
  [ModeStCalib_Pass] -> Pass/2(ModeStCalib_Pass)
  Pass/1(Pass_ArrivedTarPos) -> [Pass_ArrivedTarPos]
  [ModeStCalib_Drv] -> Drv/2(ModeStCalib_Drv)
  [DrvStConfig] -> Drv/3(StConfig)
  Drv/1(Drv_ArrivedTarPos) -> [DrvST_ArrivedTarPos]
  DrvCurPos/1 -> Drv/1(DrvCurPos)
  [DrvST_ArrivedTarPos] -> Logical Operator1/3  "LfVip_DrvST_ArrivedTarPos"
  [Pass_ArrivedTarPos] -> Logical Operator7/4  "RtVip_Pass_ArrivedTarPos"
  SecRwLtStsPossV/1 -> R2Lt/4(SecRwLtStPossV)
  DrvCurPosV/1 -> Drv/4(DrvCurPosV)
  ThdRwRtStPossV/1 -> R3Rt/4(ThdRwRtStPossV)
  SecRwRtStPossV/1 -> R2Rt/4(SecRwRtStPossV)
  PassStPossV/1 -> Pass/4(PassStPossV)
  ThdRwLtStPossV/1 -> R3Lt/4(ThdRwLtStPossV)
  Drv/2(Drv_FtUpwdDnwdPosTrgt) -> Drv_FtUpwdDnwdPosTrgt/1
  Pass/2(PassSt_FtUpwdDnwdPosTrgt) -> PassSt_FtUpwdDnwdPosTrgt/1
  PosDeltaCalib/1 -> [PosDeltaCalib]
  [PosDeltaCalib] -> Drv/5(PosDeltaCalib)
  [PosDeltaCalib] -> Pass/5(PosDeltaCalib)
  [PosDeltaCalib] -> R2Rt/5(PosDeltaCalib)
  [PosDeltaCalib] -> R2Lt/5(PosDeltaCalib)
  [PosDeltaCalib] -> R3Lt/5(PosDeltaCalib)
  [PosDeltaCalib] -> R3Rt/5(PosDeltaCalib)

== system ModeAdjust/ModeAdjustRunnable_sys/ModeAdjust/ArrivedAtTargetPosChk/Vip4s ==
  SecRwLtStsPoss : Inport
  SecRwRtStPoss : Inport  Port=2
  ModeStCalib : Inport  Port=3
  StConfig : Inport  Port=4
  SecRwLtStsPoss4s : Inport  Port=5
  SecRwRtStsPoss4s : Inport  Port=6
  StConfig4s : Inport  Port=7
  SecRwLtStsPossV : Inport  Port=8
  SecRwRtStPossV : Inport  Port=9
  SecRwLtStsPoss4sV : Inport  Port=10
  SecRwRtStsPoss4sV : Inport  Port=11
  Lt4sHightIndex : Inport  Port=12
  Rt4sHightIndex : Inport  Port=13
  PosDeltaCalib : Inport  Port=14
  Bus Selector : BusSelector  OutputSignals=Calib_Drv,Calib_Pass,Calib_2L,Calib_2R,Calib_3L,Calib_3R,Calib_2L4s,Calib_2R4s
  Bus Selector1 : BusSelector  OutputSignals=DrvStConfig,PassStConfig,SecRwLtStConfig,SecRwRtStConfig,ThdRwLtStConfig,ThdRwRtStConfig
  Bus Selector5 : BusSelector  OutputSignals=SecRwLtStConfig,SecRwRtStConfig
  R2Lt : Subsystem
  R2Rt : Subsystem
  isLfRecoveryArrivedAtTargetPos : Outport
  isRtRecoveryArrivedAtTargetPos : Outport  Port=2
  Calib_VIP4sLAdpt : Outport  Port=3
  Calib_VIP4sRAdpt : Outport  Port=4
  wires:
  [SecRwRtStConfig4s] -> R2Rt/5(StConfig4s)
  [SecRwLtStConfig4s] -> R2Lt/5(StConfig4s)
  Bus Selector5/2 -> [SecRwRtStConfig4s]  "<SecRwRtStConfig>"
  Bus Selector5/1 -> [SecRwLtStConfig4s]  "<SecRwLtStConfig>"
  StConfig4s/1 -> Bus Selector5/1
  SecRwRtStsPoss4s/1 -> R2Rt/4(SecRwLtStsPoss4s)
  SecRwLtStsPoss4s/1 -> R2Lt/4(SecRwLtStsPoss4s)
  Bus Selector/7 -> [Calib_2L4s]  "<Calib_2L4s>"
  Bus Selector/8 -> [Calib_2R4s]  "<Calib_2R4s>"
  [SecRwRtStConfig] -> R2Rt/3(StConfig)
  [SecRwLtStConfig] -> R2Lt/3(StConfig)
  Bus Selector1/5 -> [ThdRwLtStConfig]  "<ThdRwLtStConfig>"
  Bus Selector1/2 -> [PassStConfig]  "<PassStConfig>"
  StConfig/1 -> Bus Selector1/1
  Bus Selector1/4 -> [SecRwRtStConfig]  "<SecRwRtStConfig>"
  Bus Selector1/3 -> [SecRwLtStConfig]  "<SecRwLtStConfig>"
  Bus Selector1/1 -> [DrvStConfig]  "<DrvStConfig>"
  Bus Selector1/6 -> [ThdRwRtStConfig]  "<ThdRwRtStConfig>"
  [Calib_2L4s] -> R2Lt/2(ModeStCalib_2L)
  [Calib_2R4s] -> R2Rt/2(ModeStCalib_2L)
  ModeStCalib/1 -> Bus Selector/1
  Bus Selector/2 -> [ModeStCalib_Pass]  "<Calib_Pass>"
  Bus Selector/5 -> [ModeStCalib_3L]  "<Calib_3L>"
  Bus Selector/3 -> [ModeStCalib_2L]  "<Calib_2L>"
  Bus Selector/1 -> [ModeStCalib_Drv]  "<Calib_Drv>"
  Bus Selector/4 -> [ModeStCalib_2R]  "<Calib_2R>"
  Bus Selector/6 -> [ModeStCalib_3R]  "<Calib_3R>"
  [R2RtST_ArrivedTarPos] -> isRtRecoveryArrivedAtTargetPos/1
  SecRwRtStPoss/1 -> R2Rt/1(SecRwLtStsPoss)
  SecRwLtStsPoss/1 -> R2Lt/1(SecRwLtStsPoss)
  R2Rt/1(R2Lt_ArrivedTarPos) -> [R2RtST_ArrivedTarPos]
  R2Lt/1(R2Lt_ArrivedTarPos) -> [R2LtST_ArrivedTarPos]
  [R2LtST_ArrivedTarPos] -> isLfRecoveryArrivedAtTargetPos/1
  SecRwLtStsPossV/1 -> R2Lt/6(SecRwLtStPossV)
  SecRwLtStsPoss4sV/1 -> R2Lt/7(SecRwLtStPossV4s)
  SecRwRtStPossV/1 -> R2Rt/6(SecRwRtStPossV)
  SecRwRtStsPoss4sV/1 -> R2Rt/7(PosV4s)
  Lt4sHightIndex/1 -> R2Lt/8(Lt4sHightIndex)
  Rt4sHightIndex/1 -> R2Rt/8(Rt4sHightIndex)
  R2Lt/2(Calib_VIP4sLAdpt) -> Calib_VIP4sLAdpt/1
  R2Rt/2(Calib_VIP4sRAdpt) -> Calib_VIP4sRAdpt/1
  PosDeltaCalib/1 -> [PosDeltaCalib]
  [PosDeltaCalib] -> R2Lt/9(PosDeltaCalib)
  [PosDeltaCalib] -> R2Rt/9(PosDeltaCalib)

== system ModeAdjust/ModeAdjustRunnable_sys/ModeAdjust/Default/Subsystem ==
  Bus Creator2 : BusCreator  Inputs=8  OutDataTypeStr=Bus: DrvSeatPos
  PA_KeSMSwDltTrgtPos_Val{1..7,12} (8 alike) : Constant  Value=KeSMSwPosInvalidVal_Val
  DrvStTrgtPoss : Outport  VectorParamsAs1DForOutWhenUnconnected=on
  wires:
  PA_KeSMSwDltTrgtPos_Val4/1 -> Bus Creator2/5  "DrvStBkReclnUpwdDnwdTrgtPos"
  PA_KeSMSwDltTrgtPos_Val1/1 -> Bus Creator2/2  "DrvStFtUpwdDnwdTrgtPos"
  Bus Creator2/1 -> DrvStTrgtPoss/1
  PA_KeSMSwDltTrgtPos_Val6/1 -> Bus Creator2/7  "DrvStCshnRrUpwdDnwdTrgtPos"
  PA_KeSMSwDltTrgtPos_Val12/1 -> Bus Creator2/1  "DrvStBlstOtwdInwdTrgtPos"
  PA_KeSMSwDltTrgtPos_Val3/1 -> Bus Creator2/4  "DrvStLgrstUpwdDnwdTrgtPos"
  PA_KeSMSwDltTrgtPos_Val5/1 -> Bus Creator2/6  "DrvStCshnFrntUpwdDnwdTrgtPos"
  PA_KeSMSwDltTrgtPos_Val7/1 -> Bus Creator2/8  "DrvStFrwdBkwdTrgtPos"
  PA_KeSMSwDltTrgtPos_Val2/1 -> Bus Creator2/3  "DrvStHdrstUpwdDnwdTrgtPos"

== system ModeAdjust/ModeAdjustRunnable_sys/ModeAdjust/Default/Subsystem1 ==
  Bus Creator2 : BusCreator  Inputs=8  OutDataTypeStr=Bus: PasSeatPos
  PA_KeSMSwDltTrgtPos_Val{1..7,12} (8 alike) : Constant  Value=KeSMSwPosInvalidVal_Val
  PassStTrgtPoss : Outport  VectorParamsAs1DForOutWhenUnconnected=on
  wires:
  PA_KeSMSwDltTrgtPos_Val2/1 -> Bus Creator2/3  "PassStCshnFrntUpwdDnwdTrgtPos"
  PA_KeSMSwDltTrgtPos_Val1/1 -> Bus Creator2/2  "PassStBlstOtwdInwdTrgtPos"
  Bus Creator2/1 -> PassStTrgtPoss/1
  PA_KeSMSwDltTrgtPos_Val12/1 -> Bus Creator2/1  "PassStBkReclnUpwdDnwdTrgtPos"
  PA_KeSMSwDltTrgtPos_Val3/1 -> Bus Creator2/4  "PassStCshnRrUpwdDnwdTrgtPos"
  PA_KeSMSwDltTrgtPos_Val5/1 -> Bus Creator2/6  "PassStFtUpwdDnwdTrgtPos"
  PA_KeSMSwDltTrgtPos_Val7/1 -> Bus Creator2/8  "PassStLgrstUpwdDnwdTrgtPos"
  PA_KeSMSwDltTrgtPos_Val6/1 -> Bus Creator2/7  "PassStHdrstUpwdDnwdTrgtPos"
  PA_KeSMSwDltTrgtPos_Val4/1 -> Bus Creator2/5  "PassStFrwdBkwdTrgtPos"

== system ModeAdjust/ModeAdjustRunnable_sys/ModeAdjust/Default/Subsystem2 ==
  Bus Creator2 : BusCreator  Inputs=9  OutDataTypeStr=Bus: SecRwLfSeatPos
  PA_KeSMSwDltTrgtPos_Val{1..8,12} (9 alike) : Constant  Value=KeSMSwPosInvalidVal_Val
  R2Lt_TrgtPoss : Outport  VectorParamsAs1DForOutWhenUnconnected=on
  wires:
  PA_KeSMSwDltTrgtPos_Val5/1 -> Bus Creator2/6  "SecRwLtStHdrstUpwdDnwdTrgtPos"
  PA_KeSMSwDltTrgtPos_Val1/1 -> Bus Creator2/2  "SecRwLtStBlstOtwdInwdTrgtPos"
  Bus Creator2/1 -> R2Lt_TrgtPoss/1
  PA_KeSMSwDltTrgtPos_Val2/1 -> Bus Creator2/3  "SecRwLtStCshnFrntUpwdDnwdTrgtPos"
  PA_KeSMSwDltTrgtPos_Val6/1 -> Bus Creator2/7  "SecRwLtStLgrstUpwdDnwdTrgtPos"
  PA_KeSMSwDltTrgtPos_Val12/1 -> Bus Creator2/1  "SecRwLtStBkReclnUpwdDnwdTrgtPos"
  PA_KeSMSwDltTrgtPos_Val4/1 -> Bus Creator2/5  "SecRwLtStFrwdBkwdTrgtPos"
  PA_KeSMSwDltTrgtPos_Val3/1 -> Bus Creator2/4  "SecRwLtStCshnRrUpwdDnwdTrgtPos"
  PA_KeSMSwDltTrgtPos_Val7/1 -> Bus Creator2/8  "SecRwLtStLtwdRtwdTrgtPos"
  PA_KeSMSwDltTrgtPos_Val8/1 -> Bus Creator2/9  "SecRwLtStArmScrnTrgtPos"

== system ModeAdjust/ModeAdjustRunnable_sys/ModeAdjust/Default/Subsystem3 ==
  Bus Creator2 : BusCreator  Inputs=9  OutDataTypeStr=Bus: SecRwRtSeatPos
  PA_KeSMSwDltTrgtPos_Val{1..8,12} (9 alike) : Constant  Value=KeSMSwPosInvalidVal_Val
  R2Rt_TrgtPoss : Outport  VectorParamsAs1DForOutWhenUnconnected=on
  wires:
  Bus Creator2/1 -> R2Rt_TrgtPoss/1
  PA_KeSMSwDltTrgtPos_Val2/1 -> Bus Creator2/3  "SecRwRtStCshnFrntUpwdDnwdTrgtPos"
  PA_KeSMSwDltTrgtPos_Val3/1 -> Bus Creator2/4  "SecRwRtStCshnRrUpwdDnwdTrgtPos"
  PA_KeSMSwDltTrgtPos_Val4/1 -> Bus Creator2/5  "SecRwRtStFrwdBkwdTrgtPos"
  PA_KeSMSwDltTrgtPos_Val7/1 -> Bus Creator2/8  "SecRwRtStLtwdRtwdTrgtPos"
  PA_KeSMSwDltTrgtPos_Val12/1 -> Bus Creator2/1  "SecRwRtStBkReclnUpwdDnwdTrgtPos"
  PA_KeSMSwDltTrgtPos_Val6/1 -> Bus Creator2/7  "SecRwRtStLgrstUpwdDnwdTrgtPos"
  PA_KeSMSwDltTrgtPos_Val1/1 -> Bus Creator2/2  "SecRwRtStBlstOtwdInwdTrgtPos"
  PA_KeSMSwDltTrgtPos_Val5/1 -> Bus Creator2/6  "SecRwRtStHdrstUpwdDnwdTrgtPos"
  PA_KeSMSwDltTrgtPos_Val8/1 -> Bus Creator2/9  "SecRwRtStArmScrnTrgtPos"

== system ModeAdjust/ModeAdjustRunnable_sys/ModeAdjust/Default/Subsystem4 ==
  Bus Creator2 : BusCreator  Inputs=3  OutDataTypeStr=Bus: ThdRwLfSeatPos
  PA_KeSMSwDltTrgtPos_Val1 : Constant  Value=KeSMSwPosInvalidVal_Val
  PA_KeSMSwDltTrgtPos_Val12 : Constant  Value=KeSMSwPosInvalidVal_Val
  PA_KeSMSwDltTrgtPos_Val2 : Constant  Value=KeSMSwPosInvalidVal_Val
  R3Lt_TrgtPoss : Outport  VectorParamsAs1DForOutWhenUnconnected=on
  wires:
  Bus Creator2/1 -> R3Lt_TrgtPoss/1
  PA_KeSMSwDltTrgtPos_Val1/1 -> Bus Creator2/2  "ThdRwLtStCshnFldUpwdDnwdTrgtPos"
  PA_KeSMSwDltTrgtPos_Val2/1 -> Bus Creator2/3  "ThdRwLtStFrwdBkwdTrgtPos"
  PA_KeSMSwDltTrgtPos_Val12/1 -> Bus Creator2/1  "ThdRwLtStBkReclnUpwdDnwdTrgtPos"

== system ModeAdjust/ModeAdjustRunnable_sys/ModeAdjust/Default/Subsystem5 ==
  Bus Creator2 : BusCreator  Inputs=3  OutDataTypeStr=Bus: ThdRwRtSeatPos
  PA_KeSMSwDltTrgtPos_Val1 : Constant  Value=KeSMSwPosInvalidVal_Val
  PA_KeSMSwDltTrgtPos_Val2 : Constant  Value=KeSMSwPosInvalidVal_Val
  PA_KeSMSwDltTrgtPos_Val3 : Constant  Value=KeSMSwPosInvalidVal_Val
  R3Rt_TrgtPoss : Outport  VectorParamsAs1DForOutWhenUnconnected=on
  wires:
  PA_KeSMSwDltTrgtPos_Val3/1 -> Bus Creator2/3  "ThdRwRtStFrwdBkwdTrgtPos"
  Bus Creator2/1 -> R3Rt_TrgtPoss/1
  PA_KeSMSwDltTrgtPos_Val2/1 -> Bus Creator2/1  "ThdRwRtStBkReclnUpwdDnwdTrgtPos"
  PA_KeSMSwDltTrgtPos_Val1/1 -> Bus Creator2/2  "ThdRwRtStCshnFldUpwdDnwdTrgtPos"

== system ModeAdjust/ModeAdjustRunnable_sys/ModeAdjust/Default/Subsystem6 ==
  Bus Creator2 : BusCreator  Inputs=3  OutDataTypeStr=Bus: SecRwLtSt4sPos
  PA_KeSMSwDltTrgtPos_Val1 : Constant  Value=KeSMSwPosInvalidVal_Val
  PA_KeSMSwDltTrgtPos_Val2 : Constant  Value=KeSMSwPosInvalidVal_Val
  PA_KeSMSwDltTrgtPos_Val3 : Constant  Value=KeSMSwPosInvalidVal_Val
  R2Lt_TrgtPoss : Outport  VectorParamsAs1DForOutWhenUnconnected=on
  wires:
  PA_KeSMSwDltTrgtPos_Val1/1 -> Bus Creator2/2  "SecRwLtStLgrstOtwdInwdTrgtPos"
  PA_KeSMSwDltTrgtPos_Val2/1 -> Bus Creator2/1  "RrLtStFtUpwdDnwdTrgtPos"
  Bus Creator2/1 -> R2Lt_TrgtPoss/1
  PA_KeSMSwDltTrgtPos_Val3/1 -> Bus Creator2/3  "SecRwLtStHdrstFrwdBkwdTrgtPos"

== system ModeAdjust/ModeAdjustRunnable_sys/ModeAdjust/Default/Subsystem7 ==
  Bus Creator2 : BusCreator  Inputs=3  OutDataTypeStr=Bus: SecRwRtSt4sPos
  PA_KeSMSwDltTrgtPos_Val1 : Constant  Value=KeSMSwPosInvalidVal_Val
  PA_KeSMSwDltTrgtPos_Val2 : Constant  Value=KeSMSwPosInvalidVal_Val
  PA_KeSMSwDltTrgtPos_Val3 : Constant  Value=KeSMSwPosInvalidVal_Val
  R2Lt_TrgtPoss : Outport  VectorParamsAs1DForOutWhenUnconnected=on
  wires:
  Bus Creator2/1 -> R2Lt_TrgtPoss/1
  PA_KeSMSwDltTrgtPos_Val2/1 -> Bus Creator2/1  "RrRtStFtUpwdDnwdTrgtPos"
  PA_KeSMSwDltTrgtPos_Val1/1 -> Bus Creator2/2  "SecRwRtStLgrstOtwdInwdTrgtPos"
  PA_KeSMSwDltTrgtPos_Val3/1 -> Bus Creator2/3  "SecRwRtStHdrstFrwdBkwdTrgtPos"

== system ModeAdjust/ModeAdjustRunnable_sys/ModeAdjust/FAMLYL/R2Lt ==
  note: %1锁，2未锁
  note: 2L 扶手屏位置
  Mode_Trig : Inport
  Step2En : Inport  Port=2
  SecRwLtStsPoss : Inport  Port=3
  SecRwLtStPossV : Inport  Port=4
  SecRwRtStChldLkRsp_L : Inport  Port=5
  ModeStCalib_2L : Inport  Port=6
  StConfig : Inport  Port=7
  SecRwRtStChldLkRsp_R : Inport  Port=8
  Bus Creator : BusCreator  Inputs=9  OutDataTypeStr=Bus: SecRwLfSeatPos
  Bus Selector : BusSelector  OutputSignals=IfVeSMSuSecRwLtStBkReclnUpwdDnwdPos_Val_read,IfVeSMSuSecRwLtStFrwdBkwdPos_Val_read,IfVeSMSuSecRwLtStHPassStUpwdDnwdPos_Val_read,IfVeSMSuSecRwLtStLgrstUpwdDnwdPos_Val_read,IfVeSMSuSecRwLtStLtwdRtwdPos_Val_read,IfVeSMSuSecRwLtStArmScrnPos_Val_read
  Bus Selector1 : BusSelector  OutputSignals=IfVeSMSuSecRwLtStBkReclnUpwdDnwdPosV_Val_read,IfVeSMSuSecRwLtStFrwdBkwdPosV_Val_read,IfVeSMSuSecRwLtStHPassStUpwdDnwdPosV_Val_read,IfVeSMSuSecRwLtStLgrstUpwdDnwdPosV_Val_read,IfVeSMSuSecRwLtStLtwdRtwdPosV_Val_read,IfVeSMSuSecRwLtStArmScrnPosV_Val_read
  Bus Selector2 : BusSelector  OutputSignals=ArmScrnPos,ArmScrnPosMax,ArmScrnPosMin,BkReclnUpwdDnwdPos,BkReclnUpwdDnwdPosMax,BkReclnUpwdDnwdPosMin,FrwdBkwdPos,FrwdBkwdPosMax,FrwdBkwdPosMin,HdrstUpwdPos,HdrstUpwdPosMax,HdrstUpwdPosMin,LgrstUpwdPos,LgrstUpwdPosMax,LgrstUpwdPosMin,LtwdRtwdPos,LtwdRtwdPosMax,LtwdRtwdPosMin
  Bus Selector3 : BusSelector  OutputSignals=FamlyLSecRwLtSt
  Bus Selector4 : BusSelector  OutputSignals=BkReclnUpwdDnwdMovConfig,ArmTouchMovConfig,FrwdBkwdMovConfig,LgrstUpwdMovConfig,LtwdRtwdMovConfig
  Constant : Constant  Value=2  OutDataTypeStr=uint8
  Constant1 : Constant  Value=0  OutDataTypeStr=uint8
  Delay1 : Delay  DelayLength=1
  Delay2 : Delay  DelayLength=1
  Logical Operator1 : Logic  Operator=OR  AllPortsSameDT=off  OutDataTypeStr=boolean
  Logical Operator10 : Logic  Operator=OR  AllPortsSameDT=off  OutDataTypeStr=boolean
  Logical Operator2 : Logic  AllPortsSameDT=off  OutDataTypeStr=boolean
  Logical Operator3 : Logic  Operator=OR  AllPortsSameDT=off  OutDataTypeStr=boolean
  Logical Operator4 : Logic  AllPortsSameDT=off  OutDataTypeStr=boolean
  PA_KeSMSuMdMotFinshdTm_Val : Constant  Value=KeSMSuMdMotFinshdTm_Val
  PA_KeSMSuMdRetryTm1_Val : Constant  Value=KeSMSuMdRetryTm1_Val
  PA_KeSMSuModeReqDurgTm_Val : Constant  Value=KeSMSuModeReqDurgTm_Val
  PA_KeSMSuSecRwStArmTochPosDelta_Val : Constant  Value=KeSMSuSecRwStArmTochPosDelta_Val
  PA_KeSMSuSecRwStBackPosDelta_Val : Constant  Value=KeSMSuSecRwStBackPosDelta_Val
  PA_KeSMSuSecRwStFwdBkwdPosDelta_Val : Constant  Value=KeSMSuSecRwStFwdBkwdPosDelta_Val
  PA_KeSMSuSecRwStLegrestUpwdDwnwdPosDelta_Val : Constant  Value=KeSMSuSecRwStLegrestUpwdDwnwdPosDelta_Val
  PA_KeSMSuSecRwStLwdRwdPosDelta_Val : Constant  Value=KeSMSuSecRwStLwdRwdPosDelta_Val
  PA_KeSMSwDltTrgtPos_Val{1,8..9,12} (4 alike) : Constant  Value=0  OutDataTypeStr=boolean
  PA_KeSMSwDltTrgtPos_Val{3,5..7,11,14,18..21} (10 alike) : Constant  Value=KeSMSwPosInvalidVal_Val
  PA_KeSMSwDltTrgtPos_Val13 : Constant  Value=SeatChldLkSt.ChldLkSt_Unlock
  PA_KeSMSwDltTrgtPos_Val2 : Constant  Value=SeatChldLkSt.ChldLkSt_Unlock
  PA_KeSMSwDltTrgtPos_Val4 : Constant  OutDataTypeStr=boolean
  R2LtSt_FrwdBkwd_Step2_1 : Lib/CommonUsed  SystemSampleTime=-1
  R2LtSt_LtwdRtwd_Step2_2 : Lib/CommonUsed  SystemSampleTime=-1
  Relational Operator : RelationalOperator  Operator=~=  OutDataTypeStr=boolean  RndMeth=Simplest
  Relational Operator1 : RelationalOperator  Operator=~=  OutDataTypeStr=boolean  RndMeth=Simplest
  Relational Operator2 : RelationalOperator  Operator=~=  OutDataTypeStr=boolean  RndMeth=Simplest
  Switch : Switch  Criteria=u2 ~= 0
  R2Lt_Step2_Ini : Outport
  R2Lt_TrgtPoss : Outport  Port=2  VectorParamsAs1DForOutWhenUnconnected=on
  IfVeSMSuSecRwLtStRclCmdSrv_Val_writeRaw : Outport  Port=3
  R2Lt_All_done : Outport  Port=4
  R2Lt_SpdCtrl : Outport  Port=5  VectorParamsAs1DForOutWhenUnconnected=on
  wires:
  Step2En/1 -> [Step2En]
  PA_KeSMSwDltTrgtPos_Val20/1 -> Bus Creator/4  "SecRwLtStCshnRrUpwdDnwdTrgtPos"
  [R2LtStFrwdBkwd_TarPos] -> Bus Creator/5  "SecRwLtStFrwdBkwdTrgtPos"
  PA_KeSMSwDltTrgtPos_Val5/1 -> Bus Creator/1  "SecRwLtStBkReclnUpwdDnwdTrgtPos"
  PA_KeSMSwDltTrgtPos_Val18/1 -> Bus Creator/2  "SecRwLtStBlstOtwdInwdTrgtPos"
  [R2LtSt_LtwdRtwd_TarPos] -> Bus Creator/8  "SecRwLtStLtwdRtwdTrgtPos"
  PA_KeSMSwDltTrgtPos_Val19/1 -> Bus Creator/3  "SecRwLtStCshnFrntUpwdDnwdTrgtPos"
  PA_KeSMSwDltTrgtPos_Val3/1 -> Bus Creator/7  "SecRwLtStLgrstUpwdDnwdTrgtPos"
  Bus Creator/1 -> R2Lt_TrgtPoss/1
  PA_KeSMSwDltTrgtPos_Val21/1 -> Bus Creator/6  "SecRwLtStHdrstUpwdDnwdTrgtPos"
  R2LtSt_FrwdBkwd_Step2_1/2 -> [Step2_1_ArrivedTarPos]
  PA_KeSMSwDltTrgtPos_Val2/1 -> Relational Operator/2
  SecRwRtStChldLkRsp_L/1 -> Relational Operator/1
  Bus Selector/1 -> [SecRwLtStBkReclnUpwdDnwdPos]  "<IfVeSMSuSecRwLtStBkReclnUpwdDnwdPos_Val_read>"
  Bus Selector1/2 -> [SecRwLtStFrwdBkwdPosV]  "<IfVeSMSuSecRwLtStFrwdBkwdPosV_Val_read>"
  Bus Selector1/1 -> [SecRwLtStBkReclnUpwdDnwdPosV]  "<IfVeSMSuSecRwLtStBkReclnUpwdDnwdPosV_Val_read>"
  Bus Selector/2 -> [SecRwLtStFrwdBkwdPos]  "<IfVeSMSuSecRwLtStFrwdBkwdPos_Val_read>"
  Bus Selector/4 -> [SecRwLtStLgrstUpwdDnwdPos]  "<IfVeSMSuSecRwLtStLgrstUpwdDnwdPos_Val_read>"
  Bus Selector1/5 -> [SecRwLtStLtwdRtwdPosV]  "<IfVeSMSuSecRwLtStLtwdRtwdPosV_Val_read>"
  Bus Selector/3 -> [SecRwLtStHPassStUpwdDnwdPos]  "<IfVeSMSuSecRwLtStHPassStUpwdDnwdPos_Val_read>"
  SecRwLtStPossV/1 -> Bus Selector1/1
  Bus Selector1/4 -> [SecRwLtStLgrstUpwdDnwdPosV]  "<IfVeSMSuSecRwLtStLgrstUpwdDnwdPosV_Val_read>"
  SecRwLtStsPoss/1 -> Bus Selector/1
  Bus Selector/5 -> [SecRwLtStLtwdRtwdPos]  "<IfVeSMSuSecRwLtStLtwdRtwdPos_Val_read>"
  Bus Selector1/3 -> [SecRwLtStHPassStUpwdDnwdPosV]  "<IfVeSMSuSecRwLtStHPassStUpwdDnwdPosV_Val_read>"
  R2LtSt_FrwdBkwd_Step2_1/4 -> [Step2_1_done]
  R2LtSt_FrwdBkwd_Step2_1/3 -> [R2LtStFrwdBkwd_TarPos]
  [Tick] -> R2LtSt_FrwdBkwd_Step2_1/11
  PA_KeSMSwDltTrgtPos_Val6/1 -> R2LtSt_FrwdBkwd_Step2_1/10
  [SecRwLtStFrwdBkwdPosV] -> R2LtSt_FrwdBkwd_Step2_1/8
  [K_FrwdBkwdPos] -> R2LtSt_FrwdBkwd_Step2_1/6
  [Step2En] -> R2LtSt_FrwdBkwd_Step2_1/2
  [Trig] -> R2LtSt_FrwdBkwd_Step2_1/1
  R2LtSt_FrwdBkwd_Step2_1/1 -> [R2Lt_Step2_1_ini]
  [K_FrwdBkwdPosMin] -> R2LtSt_FrwdBkwd_Step2_1/4
  [KeSMSuSecRwStFwdBkwdPosDelta_Val] -> R2LtSt_FrwdBkwd_Step2_1/7
  [K_FrwdBkwdPosMax] -> R2LtSt_FrwdBkwd_Step2_1/5
  [SecRwLtStFrwdBkwdPos] -> R2LtSt_FrwdBkwd_Step2_1/3
  Mode_Trig/1 -> [Trig]
  [Step2_1_done] -> Delay1/1
  Logical Operator3/1 -> [R2Lt_Step2_1_done]
  Delay1/1 -> Logical Operator3/2
  [R2Lt_Step2_1_ini] -> Logical Operator3/1
  PA_KeSMSwDltTrgtPos_Val4/1 -> IfVeSMSuSecRwLtStRclCmdSrv_Val_writeRaw/1
  Logical Operator4/1 -> R2Lt_All_done/1
  PA_KeSMSwDltTrgtPos_Val7/1 -> Bus Creator/9  "SecRwLtStArmScrnTrgtPos"
  PA_KeSMSuSecRwStFwdBkwdPosDelta_Val/1 -> [KeSMSuSecRwStFwdBkwdPosDelta_Val]
  PA_KeSMSuSecRwStLegrestUpwdDwnwdPosDelta_Val/1 -> [KeSMSuSecRwStLegrestUpwdDwnwdPosDelta_Val]
  PA_KeSMSuSecRwStLwdRwdPosDelta_Val/1 -> [KeSMSuSecRwStLwdRwdPosDelta_Val]
  PA_KeSMSuSecRwStBackPosDelta_Val/1 -> [KeSMSuSecRwStBackPosDelta_Val]
  PA_KeSMSuMdMotFinshdTm_Val/1 -> [KeSMSuMdMotFinshdTm_Val]
  PA_KeSMSuSecRwStArmTochPosDelta_Val/1 -> [KeSMSuSecRwStArmTochPosDelta_Val]
  PA_KeSMSuModeReqDurgTm_Val/1 -> [Tick]
  [KeSMSuMdMotFinshdTm_Val] -> R2LtSt_FrwdBkwd_Step2_1/12
  Bus Selector/6 -> [SecRwLtStArmScrnPos]  "<IfVeSMSuSecRwLtStArmScrnPos_Val_read>"
  Bus Selector1/6 -> [SecRwLtStArmScrnPosV]  "<IfVeSMSuSecRwLtStArmScrnPosV_Val_read>"
  Bus Selector2/1 -> [K_ArmScrnPos]  "<ArmScrnPos>"
  Bus Selector2/18 -> [K_LtwdRtwdPosMin]  "<LtwdRtwdPosMin>"
  Bus Selector2/16 -> [K_LtwdRtwdPos]  "<LtwdRtwdPos>"
  Bus Selector2/15 -> [K_LgrstUpwdPosMin]  "<LgrstUpwdPosMin>"
  Bus Selector2/17 -> [K_LtwdRtwdPosMax]  "<LtwdRtwdPosMax>"
  Bus Selector2/12 -> [K_HdrstUpwdPosMin]  "<HdrstUpwdPosMin>"
  Bus Selector2/13 -> [K_LgrstUpwdPos]  "<LgrstUpwdPos>"
  Bus Selector2/11 -> [K_HdrstUpwdPosMax]  "<HdrstUpwdPosMax>"
  Bus Selector2/14 -> [K_LgrstUpwdPosMax]  "<LgrstUpwdPosMax>"
  Bus Selector2/10 -> [K_HdrstUpwdPos]  "<HdrstUpwdPos>"
  Bus Selector2/4 -> [K_BkReclnUpwdDnwdPos]  "<BkReclnUpwdDnwdPos>"
  Bus Selector2/9 -> [K_FrwdBkwdPosMin]  "<FrwdBkwdPosMin>"
  Bus Selector2/5 -> [K_BkReclnUpwdDnwdPosMax]  "<BkReclnUpwdDnwdPosMax>"
  Bus Selector2/8 -> [K_FrwdBkwdPosMax]  "<FrwdBkwdPosMax>"
  Bus Selector3/1 -> Bus Selector2/1  "<FamlyLSecRwLtSt>"
  Bus Selector2/7 -> [K_FrwdBkwdPos]  "<FrwdBkwdPos>"
  Bus Selector2/3 -> [K_ArmScrnPosMin]  "<ArmScrnPosMin>"
  Bus Selector2/2 -> [K_ArmScrnPosMax]  "<ArmScrnPosMax>"
  Bus Selector2/6 -> [K_BkReclnUpwdDnwdPosMin]  "<BkReclnUpwdDnwdPosMin>"
  ModeStCalib_2L/1 -> Bus Selector3/1
  PA_KeSMSwDltTrgtPos_Val8/1 -> R2LtSt_FrwdBkwd_Step2_1/13
  Bus Selector4/5 -> [LtwdRtwdMovConfig]  "<LtwdRtwdMovConfig>"
  StConfig/1 -> Bus Selector4/1
  Bus Selector4/4 -> [LgrstUpwdMovConfig]  "<LgrstUpwdMovConfig>"
  Bus Selector4/1 -> [BkReclnUpwdDnwdMovConfig]  "<BkReclnUpwdDnwdMovConfig>"
  Bus Selector4/2 -> [ArmTouchMovConfig]  "<ArmTouchMovConfig>"
  Bus Selector4/3 -> [FrwdBkwdMovConfig]  "<FrwdBkwdMovConfig>"
  [FrwdBkwdMovConfig] -> R2LtSt_FrwdBkwd_Step2_1/14
  PA_KeSMSwDltTrgtPos_Val12/1 -> R2LtSt_FrwdBkwd_Step2_1/9
  Logical Operator10/1 -> [ChildLocker]
  [KeSMSuMdMotFinshdTm_Val] -> R2LtSt_LtwdRtwd_Step2_2/12
  R2LtSt_LtwdRtwd_Step2_2/3 -> [R2LtSt_LtwdRtwd_TarPos]
  [LtwdRtwdMovConfig] -> R2LtSt_LtwdRtwd_Step2_2/14
  PA_KeSMSwDltTrgtPos_Val1/1 -> R2LtSt_LtwdRtwd_Step2_2/9
  [SecRwLtStLtwdRtwdPosV] -> R2LtSt_LtwdRtwd_Step2_2/8
  [K_LtwdRtwdPosMax] -> R2LtSt_LtwdRtwd_Step2_2/5
  R2LtSt_LtwdRtwd_Step2_2/2 -> [Step2_2_ArrivedTarPos]
  [Trig] -> R2LtSt_LtwdRtwd_Step2_2/1
  [K_LtwdRtwdPosMin] -> R2LtSt_LtwdRtwd_Step2_2/4
  PA_KeSMSwDltTrgtPos_Val14/1 -> R2LtSt_LtwdRtwd_Step2_2/10
  PA_KeSMSwDltTrgtPos_Val9/1 -> R2LtSt_LtwdRtwd_Step2_2/13
  [KeSMSuSecRwStLwdRwdPosDelta_Val] -> R2LtSt_LtwdRtwd_Step2_2/7
  [SecRwLtStLtwdRtwdPos] -> R2LtSt_LtwdRtwd_Step2_2/3
  [K_LtwdRtwdPos] -> R2LtSt_LtwdRtwd_Step2_2/6
  [Step2En] -> R2LtSt_LtwdRtwd_Step2_2/2
  R2LtSt_LtwdRtwd_Step2_2/1 -> [R2Lt_Step2_2_ini]
  R2LtSt_LtwdRtwd_Step2_2/4 -> [Step2_2_done]
  [Tick] -> R2LtSt_LtwdRtwd_Step2_2/11
  [Step2_2_done] -> Delay2/1
  Delay2/1 -> Logical Operator1/2
  [R2Lt_Step2_2_ini] -> Logical Operator1/1
  Logical Operator1/1 -> [R2Lt_Step2_2_done]
  [R2Lt_Step2_2_ini] -> Logical Operator2/2
  Logical Operator2/1 -> R2Lt_Step2_Ini/1, [R2Lt_Step2_Ini]
  [R2Lt_Step2_1_ini] -> Logical Operator2/1
  [R2Lt_Step2_1_done] -> Logical Operator4/1
  [R2Lt_Step2_2_done] -> Logical Operator4/2
  SecRwRtStChldLkRsp_R/1 -> Relational Operator1/1
  Relational Operator/1 -> Logical Operator10/1
  Relational Operator1/1 -> Logical Operator10/2
  PA_KeSMSwDltTrgtPos_Val13/1 -> Relational Operator1/2
  [CntLow] -> R2LtSt_FrwdBkwd_Step2_1/15
  [CntLow] -> R2LtSt_LtwdRtwd_Step2_2/15
  PA_KeSMSuMdRetryTm1_Val/1 -> [CntLow]
  PA_KeSMSwDltTrgtPos_Val11/1 -> Relational Operator2/2
  Constant/1 -> Switch/1
  Relational Operator2/1 -> Switch/2
  [R2LtStFrwdBkwd_TarPos] -> Relational Operator2/1
  Switch/1 -> R2Lt_SpdCtrl/1
  Constant1/1 -> Switch/3
